simulink model "Mass_est_rollfricimproved"  (R2023b)
settings: Solver=VariableStepAuto  StartTime=T_start  StopTime=T_stop  FixedStep=T_step  RelTol=1e-3
undefined symbols (not defined in the file): Aux_power, b, Batt_mdens, Battmassfrac, Crr, D, fwdorbwd, g, k, lengths, Mass, n, pground, roadcurvatures, V_end, V_start
libraries: autolibshared x2, drivinglib x1
settings Model: Creator=cas  LastModifiedBy=cas
settings DataIOCC: ExternalInput=150  ReturnWorkspaceOutputs=off  LoggingToFile=on
settings OptimizationCC: ZeroExternalMemoryAtStartup=off  ZeroInternalMemoryAtStartup=off
settings RTWCC: TargetLang=C++
settings GRTTargetCC: TargetLangStandard=C++11 (ISO)  CodeInterfacePackaging=C++ class

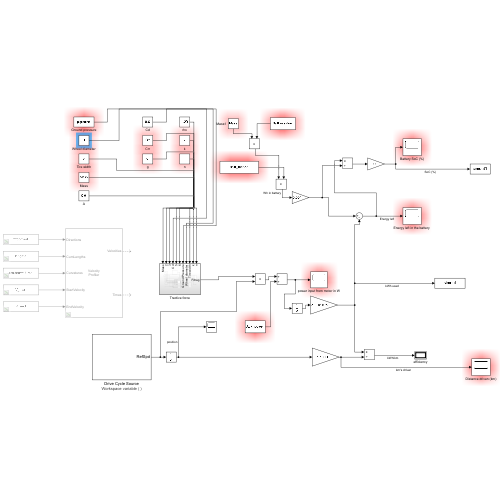
[thumbnail: Simulink's stored preview of the top-level diagram]
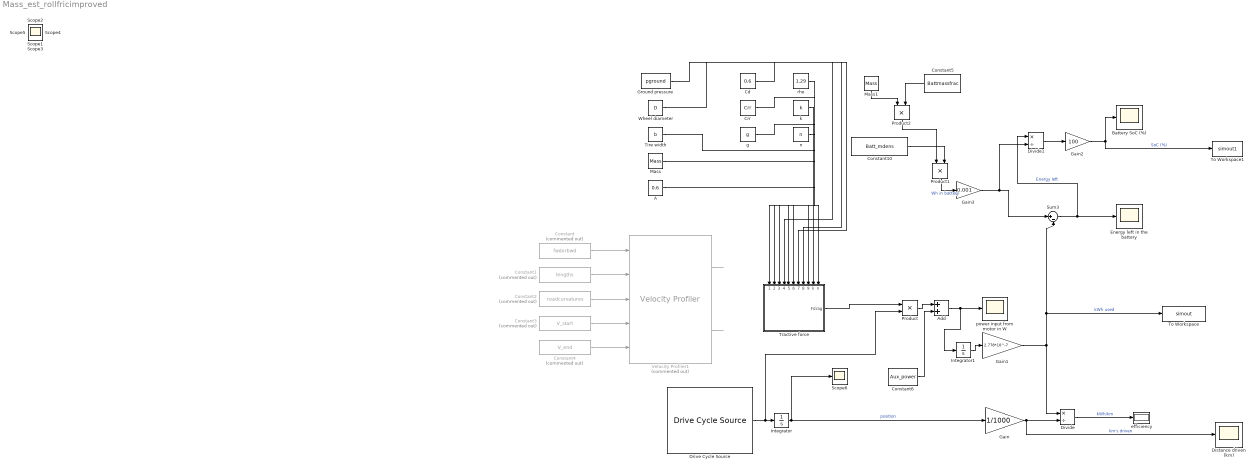
== system Mass_est_rollfricimproved ==
  A : Constant  Value=0.6
  Add : Sum
  Battery SoC (%) : Scope
  Cd : Constant  Value=0.6
  Constant : Constant  Commented=on  Value=fwdorbwd
  Constant1 : Constant  Commented=on  Value=lengths
  Constant10 : Constant  Value=Batt_mdens
  Constant2 : Constant  Commented=on  Value=roadcurvatures
  Constant3 : Constant  Commented=on  Value=V_start
  Constant4 : Constant  Commented=on  Value=V_end
  Constant5 : Constant  Value=Battmassfrac
  Constant6 : Constant  Value=Aux_power
  Crr : Constant  Value=Crr
  Distance driven (km) : Scope
  Divide : Product  Inputs=*/
  Divide1 : Product  Inputs=*/
  Drive Cycle Source : autolibshared/Drive Cycle Source  cycleVar=Workspace variable  wsVar=velocity_profile  fileVar=cycleFTP75.mat  tfinal="3070  seconds"  cycleRepeat=off  outAccPort=off  outGearPort=off  gearList=No gear data  t_wot1=5  xdot_woto=0  xdot_wot1=30  t_wot2=20  xdot_wot2=0  t_wotend=30  srcUnit=km/h  outUnit=m/s  srcAccUnit=m/s/s  outAccUnit=m/s^2  dt=0  aMode=1  faultOption=off  velBnd=2  velBndUnit=mph  inUnit=m/s  timeBnd=1  failOption=off  stopSim=off  maxFaultCnt=10  maxFaultTime=2  maxTotFaultTime=15  traceOption=off  dtTrace=1  traceWindow=10  lastDCname=Custom Data Set  lastOutUnit=mph  lastDT=0  lastTB=1  lastSB=2  forceCalcBound=off
  "Energy left in the battery " : Scope
  Gain : Gain  Gain=1/1000
  Gain1 : Gain  Gain=2.778*10^-7
  Gain2 : Gain  Gain=100
  Gain3 : Gain  Gain=0.001
  Ground pressure : Constant  Value=pground
  Integrator : Integrator
  Integrator1 : Integrator
  Mass : Constant  Value=Mass
  Mass1 : Constant  Value=Mass
  Product : Product
  Product1 : Product
  Product2 : Product
  Scope{1..6} (6 alike) : Scope
  Sum3 : Sum  Inputs=|+-
  Tire width : Constant  Value=b
  To Workspace : ToWorkspace  VariableName=simout  SampleTime=-1
      settings: Decimation=2  Save2DSignal=2-D array (concatenate along first dimension)
  To Workspace1 : ToWorkspace  VariableName=simout1  SampleTime=-1
      settings: Decimation=2  Save2DSignal=2-D array (concatenate along first dimension)
  Tractive force : Subsystem
      settings: PortSchema="{\"entries\":[{\"content\":{\"sides\":[{\"content\":{},\"type\":\"ConnectorPlacement.EquallySpacedRectSide\",\"uuid\":\"1dc941f5-3e74-4cbf-a52e-ea3cab36909e\"},{\"content\":{\"connectorIds\":[\"Out1\"],\"side\":\"RIGHT\"},\"type\":\"ConnectorPlacement.EquallySpacedRectSide\",\"uuid\":\"6f8e9dcb-b594-405f-a2b1-c41d344efafb\"},{\"content\":{\"connectorIds\":[\"In1\",\"In2\",\"In3\",\"In4\",\"In5\",\"In6\",\"In7\",\"In8\",\"In9\",\"In10\",\"In11\"],\"side\":\"TOP\"},\"type\":\"ConnectorPlacement.EquallySpacedRectSide\",\"uuid\":\"1ae95007-d3a7-4d64-89c5-5ad33b1ab93d\"}]},\"type\":\"ConnectorPlacement.EquallySpacedConnector\",\"uuid\":\"adcee74b-2e32-4cf6-bb91-c8e1408d67ea\"}],\"packageUris\":[\"http://schema.mathworks.com/mf0/Connector/R2020b\"],\"version\":\"1.0\"}"
  Velocity Profiler1 : drivinglib/Velocity Profiler  Commented=on  MaxLongitudinalAccel=3  MaxLongitudinalDecel=1  MaxSpeed=maxspeed  MaxLongitudinalJerk=1  MaxLateralAccel=1  ShowOptionalOutport=on  SampleTime=0.1  SimulateUsing=Code generation
  Wheel diameter : Constant  Value=D
  efficiency : Display
      settings: Format=bank
  g : Constant  Value=g
  k : Constant  Value=k
  n : Constant  Value=n
  power input from motor in W : Scope
  rho : Constant  Value=1.29
  wires:
  rho/1 -> Tractive force/5(In7)
  Constant3/1 -> Velocity Profiler1/4
  Constant/1 -> Velocity Profiler1/1
  Cd/1 -> Tractive force/4(Cd)
  Tractive force/1(Fdrag) -> Product/1
  g/1 -> Tractive force/2(In3)
  Constant4/1 -> Velocity Profiler1/5
  Mass/1 -> Tractive force/1(Mass)
  Velocity Profiler1/1 -> ?
  Velocity Profiler1/2 -> ?
  Integrator1/1 -> Gain1/1
  Constant1/1 -> Velocity Profiler1/2
  Divide/1 -> efficiency/1  "kWh/km"
  Gain1/1 -> Divide/1, To Workspace/1, Sum3/2  "kWh used"
  Crr/1 -> Tractive force/3(In4)
  A/1 -> Tractive force/6(In8)
  Product1/1 -> Gain3/1  "Wh in battery"
  Gain/1 -> Distance driven (km)/1, Divide/2  "km's driven"
  Constant2/1 -> Velocity Profiler1/3
  Integrator/1 -> Scope6/1, Gain/1  "position"
  Drive Cycle Source/1 -> Product/2, Integrator/1
  Constant10/1 -> Product1/2
  Sum3/1 -> Divide1/1, "Energy left in the battery "/1  "Energy left"
  Divide1/1 -> Gain2/1
  Gain2/1 -> To Workspace1/1, Battery SoC (%)/1  "SoC (%)"
  Product/1 -> Add/1
  Constant6/1 -> Add/2
  Add/1 -> Integrator1/1, power input from motor in W/1
  Mass1/1 -> Product2/1
  Constant5/1 -> Product2/2
  Product2/1 -> Product1/1
  Gain3/1 -> Divide1/2, Sum3/1
  Tire width/1 -> Tractive force/9(Tire width)
  Ground pressure/1 -> Tractive force/7(Ground Pressure)
  Wheel diameter/1 -> Tractive force/8(Wheel diameter)
  k/1 -> Tractive force/10(k)
  n/1 -> Tractive force/11(n)

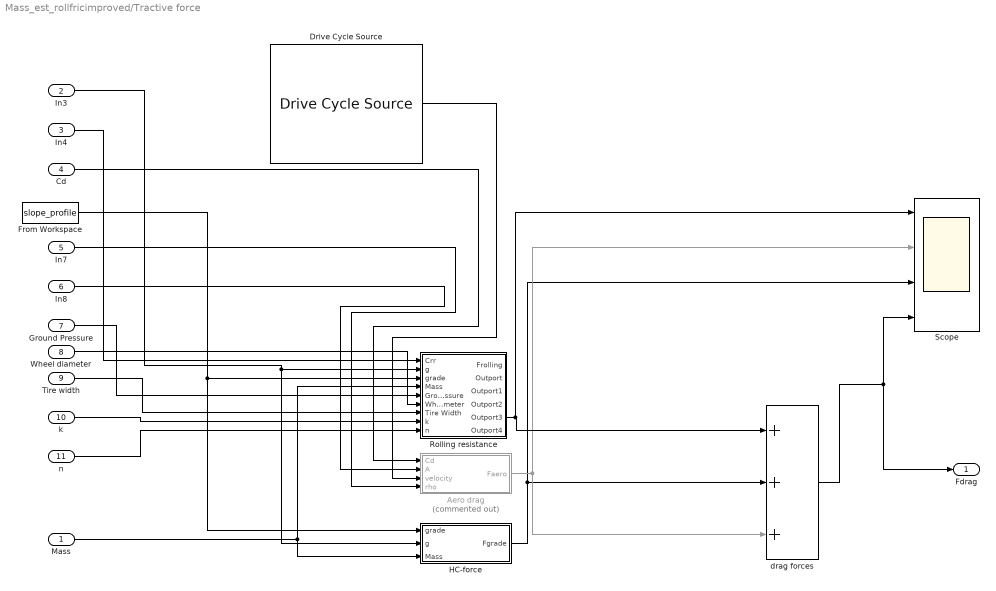
== system Mass_est_rollfricimproved/Tractive force ==
  Mass : Inport
  In3 : Inport  Port=2
  In4 : Inport  Port=3
  Cd : Inport  Port=4
  In7 : Inport  Port=5
  In8 : Inport  Port=6
  Ground Pressure : Inport  Port=7
  Wheel diameter : Inport  Port=8
  Tire width : Inport  Port=9
  k : Inport  Port=10
  n : Inport  Port=11
  Aero drag : Subsystem  Commented=on
  Drive Cycle Source : autolibshared/Drive Cycle Source  cycleVar=Workspace variable  wsVar=velocity_profile  fileVar=cycleFTP75.mat  tfinal="3070  seconds"  cycleRepeat=off  outAccPort=off  outGearPort=off  gearList=No gear data  t_wot1=5  xdot_woto=0  xdot_wot1=30  t_wot2=20  xdot_wot2=0  t_wotend=30  srcUnit=km/h  outUnit=m/s  srcAccUnit=m/s/s  outAccUnit=m/s^2  dt=0  aMode=1  faultOption=off  velBnd=2  velBndUnit=mph  inUnit=m/s  timeBnd=1  failOption=off  stopSim=off  maxFaultCnt=10  maxFaultTime=2  maxTotFaultTime=15  traceOption=off  dtTrace=1  traceWindow=10  lastDCname=Custom Data Set  lastOutUnit=mph  lastDT=0  lastTB=1  lastSB=2  forceCalcBound=off
  From Workspace : FromWorkspace  VariableName=slope_profile
  HC-force : Subsystem
  Rolling resistance : Subsystem
  Scope : Scope  NumInputPorts=4
  drag forces : Sum  Inputs=+++
  Fdrag : Outport
  wires:
  HC-force/1(Fgrade) -> Scope/3, drag forces/2
  drag forces/1 -> Fdrag/1, Scope/4
  Aero drag/1(Faero) -> Scope/2, drag forces/3
  Drive Cycle Source/1 -> Aero drag/3(velocity)
  Mass/1 -> Rolling resistance/4(Mass), HC-force/3(Mass)
  In3/1 -> HC-force/2(g), Rolling resistance/2(g)
  In4/1 -> Rolling resistance/1(Crr)
  Cd/1 -> Aero drag/1(Cd)
  From Workspace/1 -> HC-force/1(grade), Rolling resistance/3(grade)
  In7/1 -> Aero drag/4(rho)
  In8/1 -> Aero drag/2(A)
  Ground Pressure/1 -> Rolling resistance/5(Ground pressure)
  Wheel diameter/1 -> Rolling resistance/6(Wheel diameter)
  Tire width/1 -> Rolling resistance/7(Tire Width)
  k/1 -> Rolling resistance/8(k)
  n/1 -> Rolling resistance/9(n)
  Rolling resistance/5(Outport3) -> Scope/1, drag forces/1

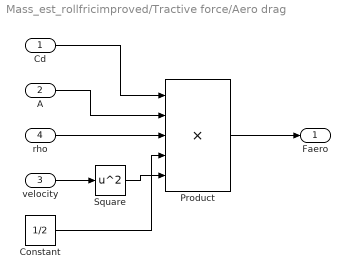
== system Mass_est_rollfricimproved/Tractive force/Aero drag ==
  Cd : Inport
  A : Inport  Port=2
  velocity : Inport  Port=3
  rho : Inport  Port=4
  Constant : Constant  Value=1/2
  Product : Product  Inputs=5
  Square : Math  Operator=square
  Faero : Outport
  wires:
  Cd/1 -> Product/1
  velocity/1 -> Square/1
  A/1 -> Product/2
  Square/1 -> Product/5
  Constant/1 -> Product/4
  Product/1 -> Faero/1
  rho/1 -> Product/3

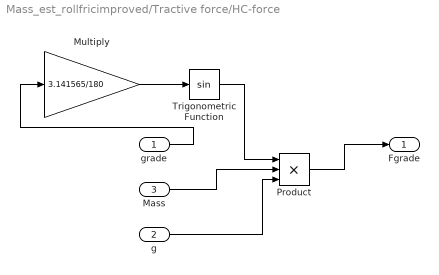
== system Mass_est_rollfricimproved/Tractive force/HC-force ==
  grade : Inport
  g : Inport  Port=2
  Mass : Inport  Port=3
  Multiply : Gain  Gain=3.141565/180
  Product : Product  Inputs=3
  Trigonometric Function : Trigonometry
  Fgrade : Outport
  wires:
  grade/1 -> Multiply/1
  Multiply/1 -> Trigonometric Function/1
  Trigonometric Function/1 -> Product/1
  Mass/1 -> Product/2
  g/1 -> Product/3
  Product/1 -> Fgrade/1

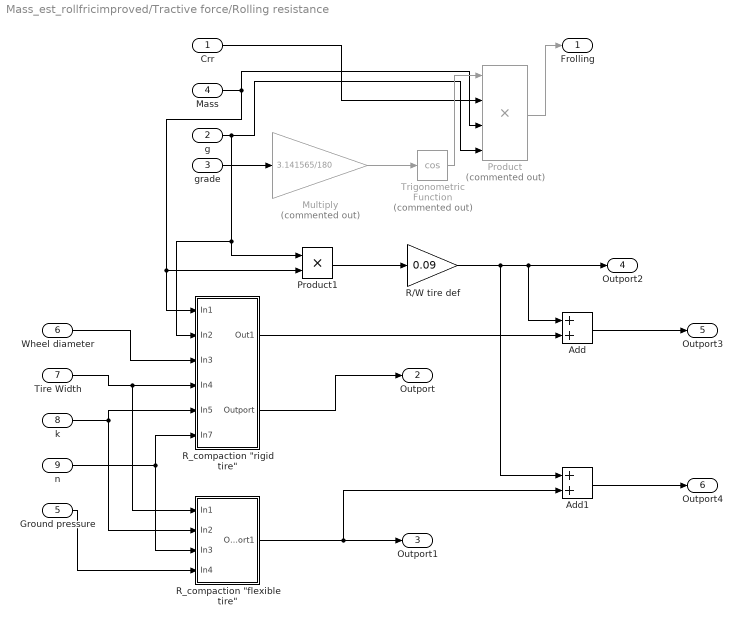
== system Mass_est_rollfricimproved/Tractive force/Rolling resistance ==
  Crr : Inport
  g : Inport  Port=2
  grade : Inport  Port=3
  Mass : Inport  Port=4
  Ground pressure : Inport  Port=5
  Wheel diameter : Inport  Port=6
  Tire Width : Inport  Port=7
  k : Inport  Port=8
  n : Inport  Port=9
  Add : Sum
  Add1 : Sum
  Multiply : Gain  Commented=on  Gain=3.141565/180
  Product : Product  Commented=on  Inputs=4
  Product1 : Product
  R/W tire def : Gain  Gain=0.09
  "R_compaction \"flexible tire\"" : Subsystem
  "R_compaction \"rigid tire\"" : Subsystem
  Trigonometric Function : Trigonometry  Commented=on  Operator=cos
  Frolling : Outport
  Outport : Outport  Port=2
  Outport1 : Outport  Port=3
  Outport2 : Outport  Port=4
  Outport3 : Outport  Port=5
  Outport4 : Outport  Port=6
  wires:
  Crr/1 -> Product/2
  Mass/1 -> "R_compaction \"rigid tire\""/1(In1), Product1/2, Product/3
  g/1 -> Product1/1, "R_compaction \"rigid tire\""/2(In2), Product/4
  grade/1 -> Multiply/1
  Multiply/1 -> Trigonometric Function/1
  Trigonometric Function/1 -> Product/1
  Product/1 -> Frolling/1
  Wheel diameter/1 -> "R_compaction \"rigid tire\""/3(In3)
  Tire Width/1 -> "R_compaction \"flexible tire\""/1(In1), "R_compaction \"rigid tire\""/4(In4)
  k/1 -> "R_compaction \"flexible tire\""/2(In2), "R_compaction \"rigid tire\""/5(In5)
  n/1 -> "R_compaction \"flexible tire\""/3(In3), "R_compaction \"rigid tire\""/6(In7)
  Ground pressure/1 -> "R_compaction \"flexible tire\""/4(In4)
  "R_compaction \"rigid tire\""/2(Outport) -> Outport/1
  "R_compaction \"flexible tire\""/1(Outport1) -> Add1/2, Outport1/1
  Product1/1 -> R/W tire def/1
  R/W tire def/1 -> Add1/1, Add/1, Outport2/1
  "R_compaction \"rigid tire\""/1(Out1) -> Add/2
  Add/1 -> Outport3/1
  Add1/1 -> Outport4/1

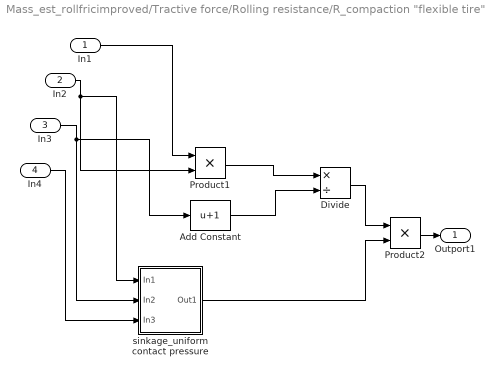
== system Mass_est_rollfricimproved/Tractive force/Rolling resistance/R_compaction "flexible tire" ==
  In1 : Inport
  In2 : Inport  Port=2
  In3 : Inport  Port=3
  In4 : Inport  Port=4
  Add Constant : Bias  Bias=1  SaturateOnIntegerOverflow=off
  Divide : Product  Inputs=*/
  Product1 : Product
  Product2 : Product
  "sinkage_uniform contact pressure " : Subsystem
  Outport1 : Outport
  wires:
  Divide/1 -> Product2/1
  Add Constant/1 -> Divide/2
  In2/1 -> "sinkage_uniform contact pressure "/1(In1), Product1/2
  Product1/1 -> Divide/1
  In3/1 -> "sinkage_uniform contact pressure "/2(In2), Add Constant/1
  In1/1 -> Product1/1
  Product2/1 -> Outport1/1
  In4/1 -> "sinkage_uniform contact pressure "/3(In3)
  "sinkage_uniform contact pressure "/1(Out1) -> Product2/2

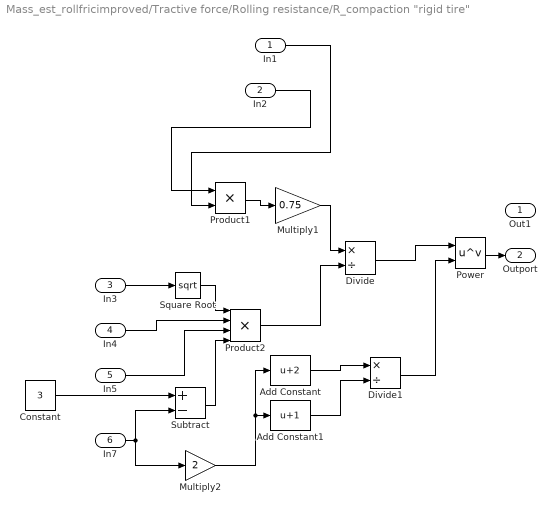
== system Mass_est_rollfricimproved/Tractive force/Rolling resistance/R_compaction "rigid tire" ==
  In1 : Inport
  In2 : Inport  Port=2
  In3 : Inport  Port=3
  In4 : Inport  Port=4
  In5 : Inport  Port=5
  In7 : Inport  Port=6
  Add Constant : Bias  Bias=2  SaturateOnIntegerOverflow=off
  Add Constant1 : Bias  Bias=1  SaturateOnIntegerOverflow=off
  Constant : Constant  Value=3
  Divide : Product  Inputs=*/  RndMeth=Zero  SaturateOnIntegerOverflow=on
  Divide1 : Product  Inputs=*/
  Multiply1 : Gain  Gain=0.75
  Multiply2 : Gain  Gain=2
  Power : Math  Operator=pow
  Product1 : Product
  Product2 : Product  Inputs=4
  Square Root : Sqrt
  Subtract : Sum  Inputs=+-
  Out1 : Outport
  Outport : Outport  Port=2
  wires:
  Square Root/1 -> Product2/1
  Divide1/1 -> Power/2
  Add Constant1/1 -> Divide1/2
  Multiply2/1 -> Add Constant1/1, Add Constant/1
  Add Constant/1 -> Divide1/1
  Subtract/1 -> Product2/4
  Product1/1 -> Multiply1/1
  Multiply1/1 -> Divide/1
  In7/1 -> Multiply2/1, Subtract/2
  Divide/1 -> Power/1
  In3/1 -> Square Root/1
  Product2/1 -> Divide/2
  In1/1 -> Product1/2
  In2/1 -> Product1/1
  In4/1 -> Product2/2
  In5/1 -> Product2/3
  Power/1 -> Outport/1
  Constant/1 -> Subtract/1

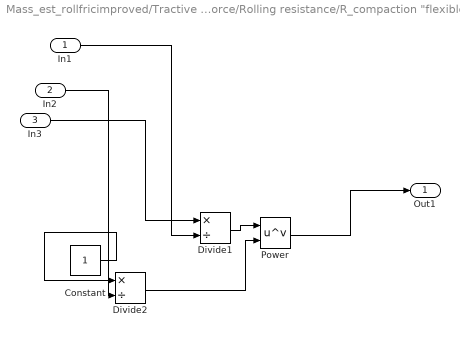
== system Mass_est_rollfricimproved/Tractive force/Rolling resistance/R_compaction "flexible tire"/sinkage_uniform contact pressure  ==
  In1 : Inport
  In2 : Inport  Port=2
  In3 : Inport  Port=3
  Constant : Constant
  Divide1 : Product  Inputs=*/
  Divide2 : Product  Inputs=*/
  Power : Math  Operator=pow
  Out1 : Outport
  wires:
  Power/1 -> Out1/1
  Divide2/1 -> Power/2
  Constant/1 -> Divide2/1
  Divide1/1 -> Power/1
  In3/1 -> Divide1/1
  In2/1 -> Divide2/2
  In1/1 -> Divide1/2
